simulink model "gm_BiSS_Splitter_Rev8"  (R2020a)
settings: Solver=FixedStepDiscrete  StartTime=0.0  StopTime=0.011  RelTol=1e-3
libraries: hdlsllib x1
settings Model: PacingRate=0.000300  Creator=asgne  LastModifiedBy=Austin
settings DataIOCC: ExternalInput=NormalSquareWave.getElement('Encoder SLO'),NormalSquareWave.getElement('DAQ Trig'),NormalSquareWave.getElement('Motor MA'),[]  LoadExternalInput=on  SaveOutput=off  SaveTime=off
settings OptimizationCC: BlockReduction=off  ConditionallyExecuteInputs=off  DefaultParameterBehavior=Inlined
settings DebuggingCC: AlgebraicLoopMsg=error  InheritedTsInSrcMsg=none  SingleTaskRateTransMsg=error
settings HardwareCC: ProdBitPerPointer=32  ProdBitPerSizeT=32  ProdBitPerPtrDiffT=32  ProdLargestAtomicFloat=None  ProdIntDivRoundTo=Undefined  ProdEndianess=Unspecified  ProdWordSize=32  ProdHWDeviceType=ASIC/FPGA->ASIC/FPGA  TargetBitPerPointer=64  TargetBitPerSizeT=64  TargetBitPerPtrDiffT=64  TargetLongLongMode=on  TargetIntDivRoundTo=Zero  TargetEndianess=LittleEndian  TargetWordSize=64  TargetHWDeviceType=Custom Processor->MATLAB Host Computer  ProdEqTarget=off

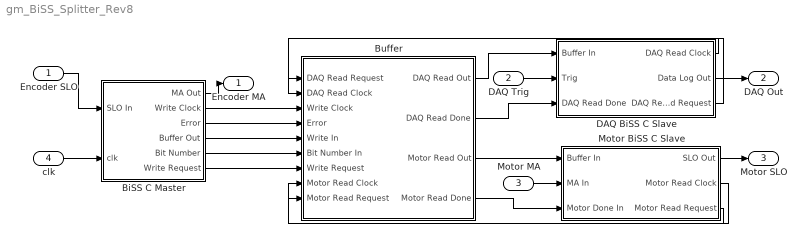
== system gm_BiSS_Splitter_Rev8 ==
  Encoder SLO : Inport  OutDataTypeStr=boolean  PortDimensions=1  SampleTime=0.00022
  DAQ Trig : Inport  Port=2  OutDataTypeStr=boolean  PortDimensions=1  SampleTime=0.00022
  Motor MA : Inport  Port=3  OutDataTypeStr=boolean  PortDimensions=1  SampleTime=0.00022
  clk : Inport  Port=4  OutDataTypeStr=boolean  PortDimensions=1  SampleTime=0.00022
  BiSS C Master : Subsystem
  Buffer : Subsystem
  DAQ BiSS C Slave : Subsystem
  Motor BiSS C Slave : Subsystem
  Encoder MA : Outport
  DAQ Out : Outport  Port=2
  Motor SLO : Outport  Port=3
  wires:
  Encoder SLO/1 -> BiSS C Master/1(SLO In)
  DAQ Trig/1 -> DAQ BiSS C Slave/2(Trig)
  Motor MA/1 -> Motor BiSS C Slave/2(MA In)
  clk/1 -> BiSS C Master/2(clk)
  BiSS C Master/1(MA Out) -> Encoder MA/1
  BiSS C Master/2(Write Clock) -> Buffer/3(Write Clock)
  BiSS C Master/3(Error) -> Buffer/4(Error)
  BiSS C Master/4(Buffer Out) -> Buffer/5(Write In)
  BiSS C Master/5(Bit Number) -> Buffer/6(Bit Number In)
  BiSS C Master/6(Write Request) -> Buffer/7(Write Request)
  Buffer/1(DAQ Read Out) -> DAQ BiSS C Slave/1(Buffer In)
  Buffer/2(DAQ Read Done) -> DAQ BiSS C Slave/3(DAQ Read Done)
  Buffer/3(Motor Read Out) -> Motor BiSS C Slave/1(Buffer In)
  Buffer/4(Motor Read Done) -> Motor BiSS C Slave/3(Motor Done In)
  DAQ BiSS C Slave/1(DAQ Read Clock) -> Buffer/2(DAQ Read Clock)
  DAQ BiSS C Slave/2(Data Log Out) -> DAQ Out/1
  DAQ BiSS C Slave/3(DAQ Read Request) -> Buffer/1(DAQ Read Request)
  Motor BiSS C Slave/1(SLO Out) -> Motor SLO/1
  Motor BiSS C Slave/2(Motor Read Clock) -> Buffer/8(Motor Read Clock)
  Motor BiSS C Slave/3(Motor Read Request) -> Buffer/9(Motor Read Request)

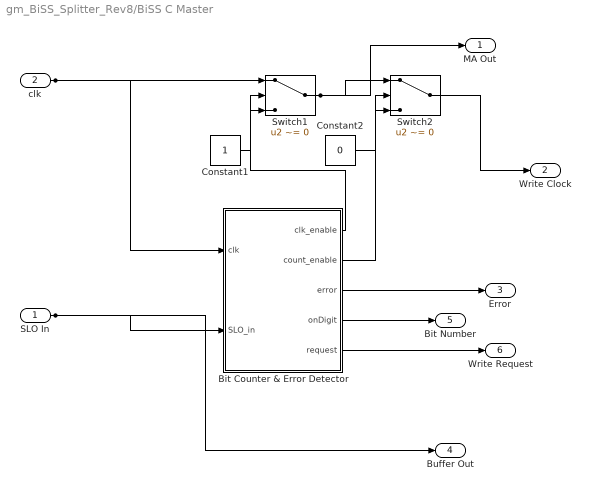
== system gm_BiSS_Splitter_Rev8/BiSS C Master ==
  SLO In : Inport  OutDataTypeStr=boolean  PortDimensions=1  SampleTime=0.00022
  clk : Inport  Port=2  OutDataTypeStr=boolean  PortDimensions=1  SampleTime=0.00022
  Bit Counter & Error Detector : Subsystem
  Constant1 : Constant  OutDataTypeStr=boolean
  Constant2 : Constant  Value=0  OutDataTypeStr=boolean
  Switch1 : Switch  Criteria=u2 ~= 0
  Switch2 : Switch  Criteria=u2 ~= 0  OutDataTypeStr=boolean
  MA Out : Outport
  Write Clock : Outport  Port=2
  Error : Outport  Port=3
  Buffer Out : Outport  Port=4
  Bit Number : Outport  Port=5
  Write Request : Outport  Port=6
  wires:
  SLO In/1 -> Bit Counter & Error Detector/2(SLO_in), Buffer Out/1
  clk/1 -> Switch1/1, Bit Counter & Error Detector/1(clk)
  Bit Counter & Error Detector/1(clk_enable) -> Switch1/2
  Bit Counter & Error Detector/2(count_enable) -> Switch2/2
  Bit Counter & Error Detector/3(error) -> Error/1
  Bit Counter & Error Detector/4(onDigit) -> Bit Number/1
  Bit Counter & Error Detector/5(request) -> Write Request/1
  Constant1/1 -> Switch1/3
  Constant2/1 -> Switch2/3
  Switch1/1 -> Switch2/1, MA Out/1
  Switch2/1 -> Write Clock/1

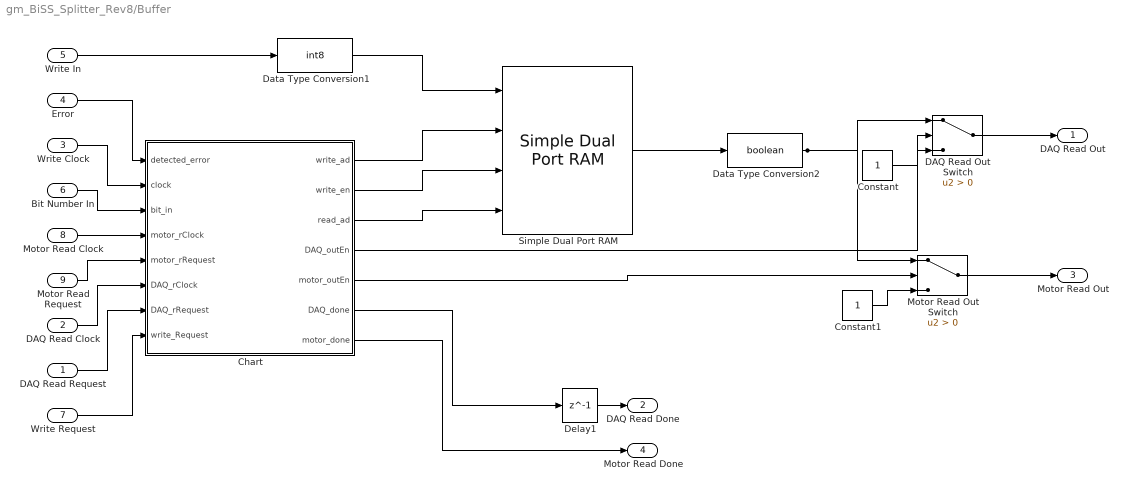
== system gm_BiSS_Splitter_Rev8/Buffer ==
  DAQ Read Request : Inport  OutDataTypeStr=boolean  PortDimensions=1  SampleTime=0.00022
  DAQ Read Clock : Inport  Port=2  OutDataTypeStr=boolean  PortDimensions=1  SampleTime=0.00022
  Write Clock : Inport  Port=3  OutDataTypeStr=boolean  PortDimensions=1  SampleTime=0.00022
  Error : Inport  Port=4  OutDataTypeStr=boolean  PortDimensions=1  SampleTime=0.00022
  Write In : Inport  Port=5  OutDataTypeStr=boolean  PortDimensions=1  SampleTime=0.00022
  Bit Number In : Inport  Port=6  OutDataTypeStr=uint8  PortDimensions=1  SampleTime=0.00022
  Write Request : Inport  Port=7  OutDataTypeStr=boolean  PortDimensions=1  SampleTime=0.00022
  Motor Read Clock : Inport  Port=8  OutDataTypeStr=boolean  PortDimensions=1  SampleTime=0.00022
  Motor Read Request : Inport  Port=9  OutDataTypeStr=boolean  PortDimensions=1  SampleTime=0.00022
  Chart : Subsystem
  Constant : Constant  OutDataTypeStr=boolean
  Constant1 : Constant  OutDataTypeStr=boolean
  DAQ Read Out Switch : Switch  Criteria=u2 > Threshold
  Data Type Conversion1 : DataTypeConversion  OutDataTypeStr=int8
  Data Type Conversion2 : DataTypeConversion  OutDataTypeStr=boolean
  Delay1 : Delay  DelayLength=1  InitialCondition=0
  Motor Read Out Switch : Switch  Criteria=u2 > Threshold
  Simple Dual Port RAM : hdlsllib/HDL RAMs/Simple Dual Port RAM  ram_size=8
      settings: SourceProductBaseCode=SL
  DAQ Read Out : Outport
  DAQ Read Done : Outport  Port=2
  Motor Read Out : Outport  Port=3
  Motor Read Done : Outport  Port=4
  wires:
  DAQ Read Request/1 -> Chart/7(DAQ_rRequest)
  DAQ Read Clock/1 -> Chart/6(DAQ_rClock)
  Write Clock/1 -> Chart/2(clock)
  Error/1 -> Chart/1(detected_error)
  Write In/1 -> Data Type Conversion1/1
  Bit Number In/1 -> Chart/3(bit_in)
  Write Request/1 -> Chart/8(write_Request)
  Motor Read Clock/1 -> Chart/4(motor_rClock)
  Motor Read Request/1 -> Chart/5(motor_rRequest)
  Chart/1(write_ad) -> Simple Dual Port RAM/2
  Chart/2(write_en) -> Simple Dual Port RAM/3
  Chart/3(read_ad) -> Simple Dual Port RAM/4
  Chart/4(DAQ_outEn) -> DAQ Read Out Switch/2
  Chart/5(motor_outEn) -> Motor Read Out Switch/2
  Chart/6(DAQ_done) -> Delay1/1
  Chart/7(motor_done) -> Motor Read Done/1
  Constant/1 -> DAQ Read Out Switch/3
  Constant1/1 -> Motor Read Out Switch/3
  DAQ Read Out Switch/1 -> DAQ Read Out/1
  Data Type Conversion1/1 -> Simple Dual Port RAM/1
  Data Type Conversion2/1 -> Motor Read Out Switch/1, DAQ Read Out Switch/1
  Delay1/1 -> DAQ Read Done/1
  Motor Read Out Switch/1 -> Motor Read Out/1
  Simple Dual Port RAM/1 -> Data Type Conversion2/1

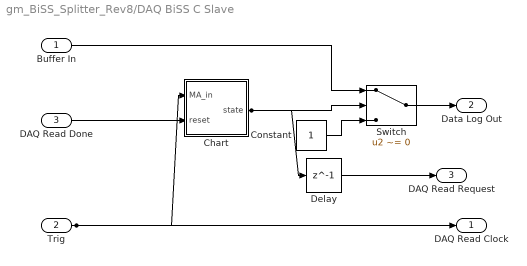
== system gm_BiSS_Splitter_Rev8/DAQ BiSS C Slave ==
  Buffer In : Inport  OutDataTypeStr=boolean  PortDimensions=1  SampleTime=0.00022
  Trig : Inport  Port=2  OutDataTypeStr=boolean  PortDimensions=1  SampleTime=0.00022
  DAQ Read Done : Inport  Port=3  OutDataTypeStr=boolean  PortDimensions=1  SampleTime=0.00022
  Chart : Subsystem
  Constant : Constant  OutDataTypeStr=boolean
  Delay : Delay  DelayLength=1  InitialCondition=0
  Switch : Switch  Criteria=u2 ~= 0
  DAQ Read Clock : Outport
  Data Log Out : Outport  Port=2
  DAQ Read Request : Outport  Port=3
  wires:
  Buffer In/1 -> Switch/1
  Trig/1 -> Chart/1(MA_in), DAQ Read Clock/1
  DAQ Read Done/1 -> Chart/2(reset)
  Chart/1(state) -> Switch/2, Delay/1
  Constant/1 -> Switch/3
  Delay/1 -> DAQ Read Request/1
  Switch/1 -> Data Log Out/1

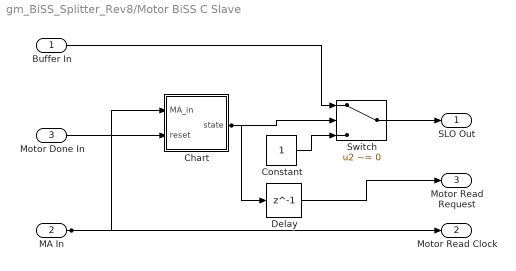
== system gm_BiSS_Splitter_Rev8/Motor BiSS C Slave ==
  Buffer In : Inport  OutDataTypeStr=boolean  PortDimensions=1  SampleTime=0.00022
  MA In : Inport  Port=2  OutDataTypeStr=boolean  PortDimensions=1  SampleTime=0.00022
  Motor Done In : Inport  Port=3  OutDataTypeStr=boolean  PortDimensions=1  SampleTime=0.00022
  Chart : Subsystem
  Constant : Constant  OutDataTypeStr=boolean
  Delay : Delay  DelayLength=1  InitialCondition=0
  Switch : Switch  Criteria=u2 ~= 0
  SLO Out : Outport
  Motor Read Clock : Outport  Port=2
  Motor Read Request : Outport  Port=3
  wires:
  Buffer In/1 -> Switch/1
  MA In/1 -> Chart/1(MA_in), Motor Read Clock/1
  Motor Done In/1 -> Chart/2(reset)
  Chart/1(state) -> Switch/2, Delay/1
  Constant/1 -> Switch/3
  Delay/1 -> Motor Read Request/1
  Switch/1 -> SLO Out/1

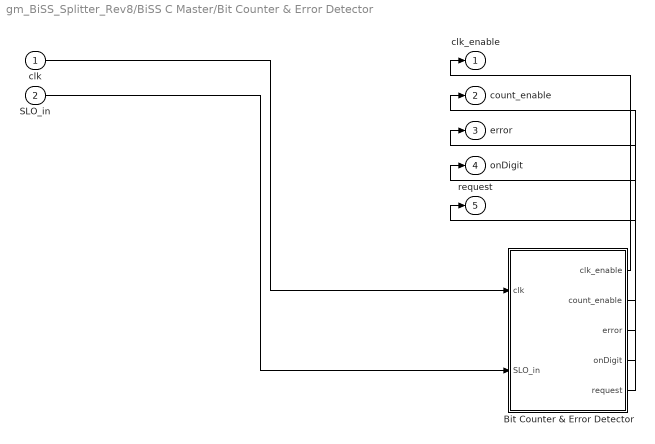
== system gm_BiSS_Splitter_Rev8/BiSS C Master/Bit Counter & Error Detector ==
  clk : Inport  OutDataTypeStr=boolean  PortDimensions=1  SampleTime=0.00022
  SLO_in : Inport  Port=2  OutDataTypeStr=boolean  PortDimensions=1  SampleTime=0.00022
  Bit Counter & Error Detector : Stateflow chart  TreatAsAtomicUnit=on
  clk_enable : Outport
  count_enable : Outport  Port=2
  error : Outport  Port=3
  onDigit : Outport  Port=4
  request : Outport  Port=5
  wires:
  clk/1 -> Bit Counter & Error Detector/1(clk)
  SLO_in/1 -> Bit Counter & Error Detector/2(SLO_in)
  Bit Counter & Error Detector/1(clk_enable) -> clk_enable/1
  Bit Counter & Error Detector/2(count_enable) -> count_enable/1
  Bit Counter & Error Detector/3(error) -> error/1
  Bit Counter & Error Detector/4(onDigit) -> onDigit/1
  Bit Counter & Error Detector/5(request) -> request/1

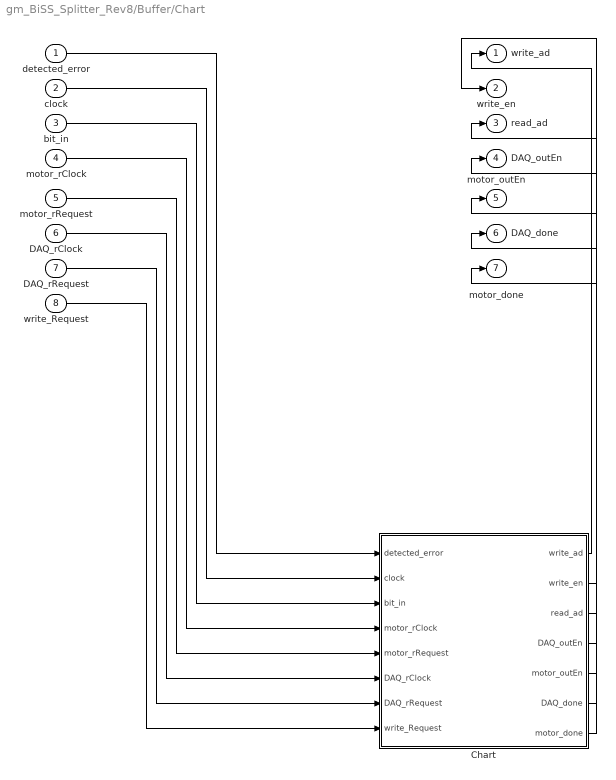
== system gm_BiSS_Splitter_Rev8/Buffer/Chart ==
  detected_error : Inport  OutDataTypeStr=boolean  PortDimensions=1  SampleTime=0.00022
  clock : Inport  Port=2  OutDataTypeStr=boolean  PortDimensions=1  SampleTime=0.00022
  bit_in : Inport  Port=3  OutDataTypeStr=uint8  PortDimensions=1  SampleTime=0.00022
  motor_rClock : Inport  Port=4  OutDataTypeStr=boolean  PortDimensions=1  SampleTime=0.00022
  motor_rRequest : Inport  Port=5  OutDataTypeStr=boolean  PortDimensions=1  SampleTime=0.00022
  DAQ_rClock : Inport  Port=6  OutDataTypeStr=boolean  PortDimensions=1  SampleTime=0.00022
  DAQ_rRequest : Inport  Port=7  OutDataTypeStr=boolean  PortDimensions=1  SampleTime=0.00022
  write_Request : Inport  Port=8  OutDataTypeStr=boolean  PortDimensions=1  SampleTime=0.00022
  Chart : Stateflow chart  TreatAsAtomicUnit=on
  write_ad : Outport
  write_en : Outport  Port=2
  read_ad : Outport  Port=3
  DAQ_outEn : Outport  Port=4
  motor_outEn : Outport  Port=5
  DAQ_done : Outport  Port=6
  motor_done : Outport  Port=7
  wires:
  detected_error/1 -> Chart/1(detected_error)
  clock/1 -> Chart/2(clock)
  bit_in/1 -> Chart/3(bit_in)
  motor_rClock/1 -> Chart/4(motor_rClock)
  motor_rRequest/1 -> Chart/5(motor_rRequest)
  DAQ_rClock/1 -> Chart/6(DAQ_rClock)
  DAQ_rRequest/1 -> Chart/7(DAQ_rRequest)
  write_Request/1 -> Chart/8(write_Request)
  Chart/1(write_ad) -> write_ad/1
  Chart/2(write_en) -> write_en/1
  Chart/3(read_ad) -> read_ad/1
  Chart/4(DAQ_outEn) -> DAQ_outEn/1
  Chart/5(motor_outEn) -> motor_outEn/1
  Chart/6(DAQ_done) -> DAQ_done/1
  Chart/7(motor_done) -> motor_done/1

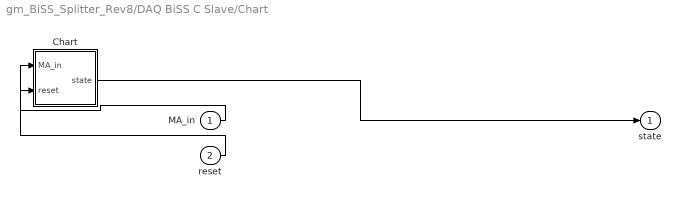
== system gm_BiSS_Splitter_Rev8/DAQ BiSS C Slave/Chart ==
  MA_in : Inport  OutDataTypeStr=boolean  PortDimensions=1  SampleTime=0.00022
  reset : Inport  Port=2  OutDataTypeStr=boolean  PortDimensions=1  SampleTime=0.00022
  Chart : Stateflow chart  TreatAsAtomicUnit=on
  state : Outport
  wires:
  MA_in/1 -> Chart/1(MA_in)
  reset/1 -> Chart/2(reset)
  Chart/1(state) -> state/1

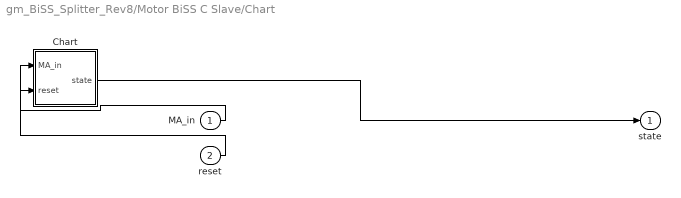
== system gm_BiSS_Splitter_Rev8/Motor BiSS C Slave/Chart ==
  MA_in : Inport  OutDataTypeStr=boolean  PortDimensions=1  SampleTime=0.00022
  reset : Inport  Port=2  OutDataTypeStr=boolean  PortDimensions=1  SampleTime=0.00022
  Chart : Stateflow chart  TreatAsAtomicUnit=on
  state : Outport
  wires:
  Chart/1(state) -> state/1
  reset/1 -> Chart/2(reset)
  MA_in/1 -> Chart/1(MA_in)

== stateflow chart gm_BiSS_Splitter_Rev8/DAQ BiSS C Slave/Chart/Chart ==
  settings: executeAtInitialization=1
  state Off
    state = false;
  state On
    state = true;
  (default) -> Off
  Off -> On : [MA_in == false]
  On -> Off : [reset == true && MA_in == true]
  data: MA_in input; reset input; state output

== stateflow chart gm_BiSS_Splitter_Rev8/BiSS C Master/Bit Counter & Error Detector/Bit Counter & Error Detector ==
  settings: executeAtInitialization=1
  note: This state diagram runs in circles to determine which part of the BiSS C waveform
      | the splitter is currently recieving, and make appropriate actions based off of that.
  state Ready
    entry: count_enable = false;
    request = false;
  state Ack
    entry:
    error = false;
    clk_enable = true;
    request= true;
  state Start
  state Zero
  state Read
    entry:
    clk_enable = true;
    keeper = int8(1);
    onDigit = uint8(1);
    count_enable = true;
    counter = uint8(1);
    errorKeeper = false;
    during:
    if clk == true && keeper == 0
    counter = counter +1;
    keeper = 1;
    if counter < 43
    onDigit = counter;
    else
    onDigit = 0;
    clk_enable=false;
    end
    elseif clk == false
    keeper = 0;
    end
    if onDigit == 33 && errorKeeper == false
    if SLO_in == 1
    error = true;
    end
    errorKeeper = true;
    end
    exit: onDigit =0;
    clk_enable = false;
    request = false
  (default) -> Ready
  Read -> Ready : [counter == 43 && clk == true]
  Ready -> Ack : [SLO_in == true && clk == true]
  Ack -> Start : [SLO_in == false && clk == true]
  Start -> Zero : [SLO_in == true && clk == true]
  Zero -> Read : [SLO_in==false && clk == true]
  data: clk input; SLO_in input; clk_enable output boolean; count_enable output boolean; error output boolean; keeper local; onDigit output uint8; request output boolean; errorKeeper local boolean; counter local

== stateflow chart gm_BiSS_Splitter_Rev8/Motor BiSS C Slave/Chart/Chart ==
  settings: executeAtInitialization=1
  state Off
    state = false;
  state On
    state = true;
  (default) -> Off
  Off -> On : [MA_in == false]
  On -> Off : [reset == true && MA_in == true]
  data: MA_in input; reset input; state output

== stateflow chart gm_BiSS_Splitter_Rev8/Buffer/Chart/Chart ==
  settings: executeAtInitialization=1
  state Initialization
    entry: bankToggle1 = 0;
    bankToggle2 = 1;
  state MotorRead
    entry:
    read_keeper = 0;
    onDigit_read = 0;
    motor_outEn = true;
    during:
    if motor_rClock == true && read_keeper == 0 && onDigit_read <42
    onDigit_read = onDigit_read +1;
    read_keeper = 1;
    elseif motor_rClock == false
    read_keeper = 0;
    else
    end
    read_ad = onDigit_read + (bankToggle2*50);
    exit: motor_done = true;
    motor_outEn = false;
    read_ad = 0;
  state DAQRead
    entry:
    read_keeper = 0;
    onDigit_read = 0;
    DAQ_outEn = true;
    during:
    if DAQ_rClock == true && read_keeper == 0 && onDigit_read <42
    onDigit_read = onDigit_read +1;
    read_keeper = 1;
    elseif DAQ_rClock == false
    read_keeper = 0;
    else
    end
    read_ad = onDigit_read + (bankToggle2*50);
    exit: DAQ_done = true;
    DAQ_outEn = false
    read_ad = 0;
  state NormalOperation
    exit:
    motor_done = false;
    DAQ_done = false;
  state MotorReadandWrite
    entry:
    read_keeper = 0;
    onDigit_read = 0;
    write_keeper = false;
    write_ad = bit_in + (bankToggle1*50);
    motor_outEn = true;
    if clock == true
    write_en = true;
    else
    write_en = false;
    end
    during:
    if motor_rClock == true && read_keeper == 0 && onDigit_read<42
    onDigit_read = onDigit_read +1;
    read_keeper = 1;
    elseif motor_rClock == false
    read_keeper = 0;
    end
    read_ad = onDigit_read + (bankToggle2*50);
    if bit_in == 0
    write_keeper = true;
    write_ad = 0;
    end
    if write_keeper == false
    write_ad = bit_in + (bankToggle1*50);
    end
    if clock == true && write_keeper == false
    write_en = true;
    else
    write_en = false;
    end
    exit: motor_done = true;
    motor_outEn = false;
    write_en = false;
    write_ad =0;
    read_ad = 0;
  state DAQReadandWrite
    entry:
    read_keeper = 0;
    onDigit_read = 0;
    write_keeper = false;
    write_ad = bit_in + (bankToggle1*50);
    motor_outEn = true;
    if clock == true
    write_en = true;
    else
    write_en = false;
    end
    during:
    if DAQ_rClock == true && read_keeper == 0 && onDigit_read<42
    onDigit_read = onDigit_read +1;
    read_keeper = 1;
    elseif DAQ_rClock == false
    read_keeper = 0;
    end
    read_ad = onDigit_read + (bankToggle2*50);
    if bit_in == 0
    write_keeper = true;
    write_ad = 0;
    end
    if write_keeper == false
    write_ad = bit_in + (bankToggle1*50);
    end
    if clock == true && write_keeper == false
    write_en = true;
    else
    write_en = false;
    end
    exit: motor_done = true;
    motor_outEn = false;
    write_en = false;
    write_ad =0;
    read_ad = 0;
  state WriteOnly
    entry:
    write_ad = bit_in + (bankToggle1*50);
    if clock == true
    write_en = true
    else
    write_en = false
    end
    during:
    write_ad = bit_in + (bankToggle1*50);
    if clock == true
    write_en = true
    else
    write_en = false
    end
    exit: write_en = false;
    write_ad =0;
  state SwitchBank
    exit:
    if detected_error == false
    if bankToggle1 == 0
    bankToggle1 = 1;
    bankToggle2 = 0;
    else
    bankToggle1 = 0;
    bankToggle2 = 1;
    end
    end
  (default) -> Initialization
  Initialization -> NormalOperation
  DAQRead -> NormalOperation : [onDigit_read ==42 && motor_rClock == false]
  MotorRead -> NormalOperation : [onDigit_read == 42 && motor_rClock == false ]
  NormalOperation -> MotorRead [order 2] : [motor_rRequest ==true && write_Request == false]
  NormalOperation -> DAQRead [order 4] : [DAQ_rRequest ==true && write_Request == false]
  NormalOperation -> MotorReadandWrite [order 1] : [motor_rRequest ==true && write_Request ==true && bit_in == 1]
  NormalOperation -> DAQReadandWrite [order 3] : [DAQ_rRequest ==true && write_Request ==true && bit_in == 1]
  SwitchBank -> NormalOperation
  NormalOperation -> WriteOnly [order 5] : [write_Request ==true && bit_in == 1]
  WriteOnly -> SwitchBank : [bit_in == 0]
  DAQReadandWrite -> SwitchBank : [bit_in == 0 && onDigit_read == 42]
  MotorReadandWrite -> SwitchBank : [bit_in == 0 && onDigit_read == 42]
  data: detected_error input boolean; clock input boolean; bit_in input uint8; motor_rClock input boolean; motor_rRequest input boolean; DAQ_rClock input boolean; write_ad output uint8; write_en output boolean; read_ad output uint8; DAQ_outEn output boolean; motor_outEn output boolean; DAQ_done output boolean; motor_done output boolean; bankToggle2 local uint8; bankToggle1 local uint8; onDigit_read local uint8; read_keeper local int8; DAQ_rRequest input boolean; write_Request input; write_keeper local
